simulink model "ThdRwLtStFwdBkwdCtrl"  (R2024b)
settings: Solver=FixedStepDiscrete  StartTime=0.0  StopTime=10.0  FixedStep=0.01  RelTol=1e-3
undefined symbols (not defined in the file or in its folder): KeSMSuMdMotFinshdTm_Val, KeSMSuMdRetryTm1_Val, KeSMSuModeReqDurgTm_Val, KeSMSwThdRwLtStFwdBkwdEnTrigBitMask6s_Val, KeSMSwThdRwLtStFwdBkwdEnTrigBitMask_Val
libraries: StCtrlLibBkRecln x1
settings Model: ModifiedHistory=24.6.21 V2.4.0 557模式流程V1.6  Creator=sn2xws  LastModifiedBy=sn55gm
settings SolverCC: AlgebraicLoopSolver=TrustRegion
settings DataIOCC: SaveFormat=StructureWithTime  ReturnWorkspaceOutputs=off
settings OptimizationCC: DefaultParameterBehavior=Inlined  EnhancedBackFolding=on  PassReuseOutputArgsAs=Individual arguments  ZeroExternalMemoryAtStartup=off  ZeroInternalMemoryAtStartup=off  OptimizeBlockOrder=speed  DifferentSizesBufferReuse=on  OptimizationCustomize=off  EfficientTunableParamExpr=on
settings DebuggingCC: ParameterTunabilityLossMsg=error  UnconnectedInputMsg=warning  UnconnectedOutputMsg=warning  UnconnectedLineMsg=warning  ArithmeticOperatorsInVariantConditions=warning
settings ModelReferenceCC: EnableRefExpFcnMdlSchedulingChecks=on  ModelReferenceNumInstancesAllowed=Single
settings SFSimCC: MATLABDynamicMemAlloc=off  CustomCodeUndefinedFunction=UseInterfaceOnly
settings RTWCC: Description=AUTOSAR  SystemTargetFile=autosar.tlc  GenCodeOnly=on  TemplateMakefile=ert_default_tmf  GenerateReport=on  IncludeHyperlinkInReport=on  LaunchReport=on  DataTypeReplacement=CDataTypesFixedWidth  GenerateTraceInfo=on  GenerateTraceReport=on  GenerateTraceReportSl=on  GenerateTraceReportSf=on  GenerateTraceReportEml=on  GPUComputeCapability=3.5
settings CodeAppCC: ForceParamTrailComments=on  IgnoreCustomStorageClasses=off  OperatorAnnotations=on  SimulinkDataObjDesc=on  SFDataObjDesc=on  InsertBlockDesc=on
settings STFCustomTargetCC: TargetLangStandard=C99 (ISO)  MultiwordLength=256  ParMdlRefBuildCompliant=on  CompOptLevelCompliant=on  IncludeMdlTerminateFcn=off  CombineOutputUpdateFcns=on  SuppressErrorStatus=on  ERTCustomFileBanners=on  SupportNonFinite=off  SupportComplex=off  SupportContinuousTime=off  SupportNonInlinedSFcns=off  RemoveResetFunc=on  MATLABClassNameForMDSCustomization=Simulink.SoftwareTarget.ERTCustomization  AutosarCompliant=on  UseToolchainInfoCompliant=on  LookupTableObjectStructAxisOrder=2,1,3,4,...  LUTObjectStructOrderEvenSpacing=Size,Table,Breakpoints  SystemTargetFile=autosar.tlc
settings ERTTargetCC: TargetLangStandard=C99 (ISO)  ConcurrentExecutionCompliant=off  IncludeMdlTerminateFcn=off  SuppressErrorStatus=on  SupportNonFinite=off  SupportComplex=off  ModelStepFunctionPrototypeControlCompliant=off  CPPClassGenCompliant=off  AutosarCompliant=on  LookupTableObjectStructAxisOrder=2,1,3,4,...  LUTObjectStructOrderEvenSpacing=Size,Table,Breakpoints  ERTCustomFileTemplate=example_file_process.tlc  ERTFilePackagingFormat=Compact  BooleanTrueId=TRUE  BooleanFalseId=FALSE  DynamicArrayContainerType=coder::array

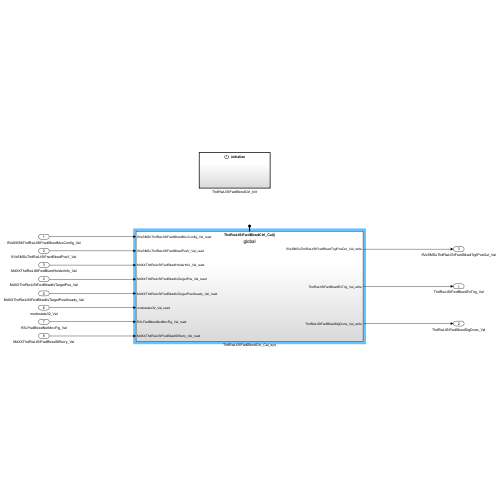
[thumbnail: Simulink's stored preview of the top-level diagram]
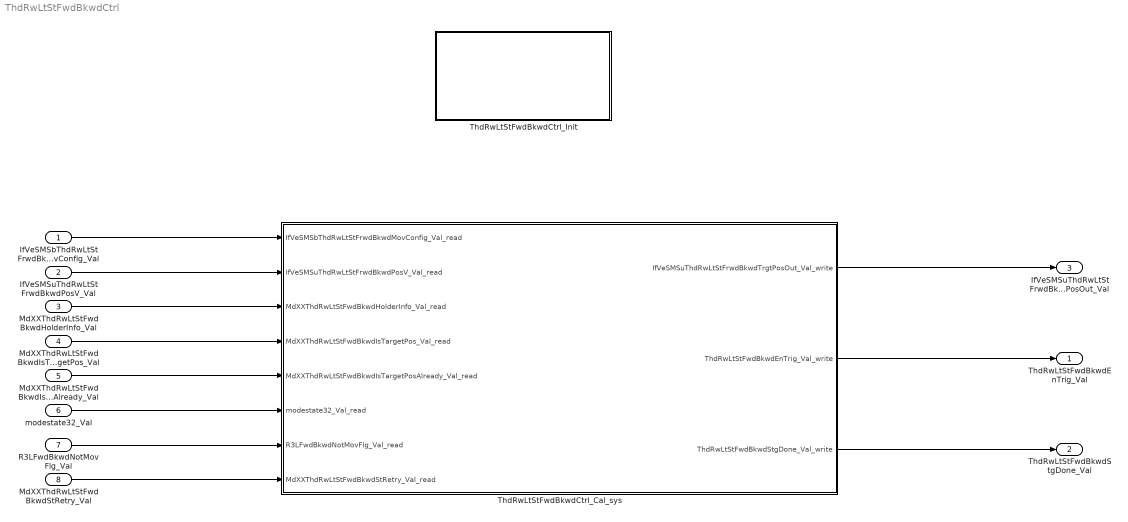
== system ThdRwLtStFwdBkwdCtrl ==
  IfVeSMSbThdRwLtStFrwdBkwdMovConfig_Val : Inport  OutDataTypeStr=boolean  PortDimensions=1
  IfVeSMSuThdRwLtStFrwdBkwdPosV_Val : Inport  Port=2  OutDataTypeStr=boolean  PortDimensions=1
  MdXXThdRwLtStFwdBkwdHolderInfo_Val : Inport  Port=3  OutDataTypeStr=uint32  PortDimensions=1
  MdXXThdRwLtStFwdBkwdIsTargetPos_Val : Inport  Port=4  OutDataTypeStr=uint32  PortDimensions=1
  MdXXThdRwLtStFwdBkwdIsTargetPosAlready_Val : Inport  Port=5  OutDataTypeStr=uint32  PortDimensions=1
  modestate32_Val : Inport  Port=6  OutDataTypeStr=uint32  PortDimensions=1
  R3LFwdBkwdNotMovFlg_Val : Inport  Port=7  OutDataTypeStr=boolean  PortDimensions=1
  MdXXThdRwLtStFwdBkwdStRetry_Val : Inport  Port=8  OutDataTypeStr=uint32  PortDimensions=1
  ThdRwLtStFwdBkwdCtrl_Cal_sys : Subsystem
  ThdRwLtStFwdBkwdCtrl_Init : Subsystem
  ThdRwLtStFwdBkwdEnTrig_Val : Outport  OutDataTypeStr=boolean  PortDimensions=1  VectorParamsAs1DForOutWhenUnconnected=off
  ThdRwLtStFwdBkwdStgDone_Val : Outport  Port=2  OutDataTypeStr=boolean  PortDimensions=1  VectorParamsAs1DForOutWhenUnconnected=off
  IfVeSMSuThdRwLtStFrwdBkwdTrgtPosOut_Val : Outport  Port=3  OutDataTypeStr=boolean  PortDimensions=1  VectorParamsAs1DForOutWhenUnconnected=off
  wires:
  IfVeSMSbThdRwLtStFrwdBkwdMovConfig_Val/1 -> ThdRwLtStFwdBkwdCtrl_Cal_sys/1(IfVeSMSbThdRwLtStFrwdBkwdMovConfig_Val_read)
  IfVeSMSuThdRwLtStFrwdBkwdPosV_Val/1 -> ThdRwLtStFwdBkwdCtrl_Cal_sys/2(IfVeSMSuThdRwLtStFrwdBkwdPosV_Val_read)
  MdXXThdRwLtStFwdBkwdHolderInfo_Val/1 -> ThdRwLtStFwdBkwdCtrl_Cal_sys/3(MdXXThdRwLtStFwdBkwdHolderInfo_Val_read)
  MdXXThdRwLtStFwdBkwdIsTargetPos_Val/1 -> ThdRwLtStFwdBkwdCtrl_Cal_sys/4(MdXXThdRwLtStFwdBkwdIsTargetPos_Val_read)
  MdXXThdRwLtStFwdBkwdIsTargetPosAlready_Val/1 -> ThdRwLtStFwdBkwdCtrl_Cal_sys/5(MdXXThdRwLtStFwdBkwdIsTargetPosAlready_Val_read)
  modestate32_Val/1 -> ThdRwLtStFwdBkwdCtrl_Cal_sys/6(modestate32_Val_read)
  R3LFwdBkwdNotMovFlg_Val/1 -> ThdRwLtStFwdBkwdCtrl_Cal_sys/7(R3LFwdBkwdNotMovFlg_Val_read)
  ThdRwLtStFwdBkwdCtrl_Cal_sys/1(IfVeSMSuThdRwLtStFrwdBkwdTrgtPosOut_Val_write) -> IfVeSMSuThdRwLtStFrwdBkwdTrgtPosOut_Val/1
  ThdRwLtStFwdBkwdCtrl_Cal_sys/2(ThdRwLtStFwdBkwdEnTrig_Val_write) -> ThdRwLtStFwdBkwdEnTrig_Val/1
  ThdRwLtStFwdBkwdCtrl_Cal_sys/3(ThdRwLtStFwdBkwdStgDone_Val_write) -> ThdRwLtStFwdBkwdStgDone_Val/1
  MdXXThdRwLtStFwdBkwdStRetry_Val/1 -> ThdRwLtStFwdBkwdCtrl_Cal_sys/8(MdXXThdRwLtStFwdBkwdStRetry_Val_read)

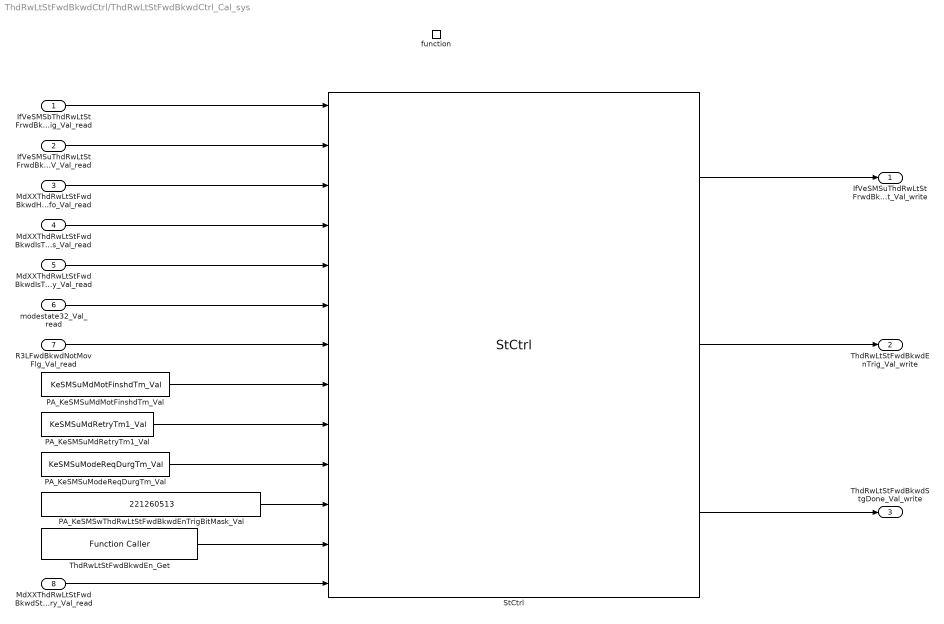
== system ThdRwLtStFwdBkwdCtrl/ThdRwLtStFwdBkwdCtrl_Cal_sys ==
  IfVeSMSbThdRwLtStFrwdBkwdMovConfig_Val_read : Inport
  IfVeSMSuThdRwLtStFrwdBkwdPosV_Val_read : Inport  Port=2
  MdXXThdRwLtStFwdBkwdHolderInfo_Val_read : Inport  Port=3
  MdXXThdRwLtStFwdBkwdIsTargetPos_Val_read : Inport  Port=4
  MdXXThdRwLtStFwdBkwdIsTargetPosAlready_Val_read : Inport  Port=5
  modestate32_Val_read : Inport  Port=6
  R3LFwdBkwdNotMovFlg_Val_read : Inport  Port=7
  MdXXThdRwLtStFwdBkwdStRetry_Val_read : Inport  Port=8
  function : TriggerPort  TriggerType=function-call  IsSimulinkFunction=on  FunctionName=ThdRwLtStFwdBkwdCtrl_Cal  VariantControl=(inherit)
  PA_KeSMSuMdMotFinshdTm_Val : Constant  Value=KeSMSuMdMotFinshdTm_Val
  PA_KeSMSuMdRetryTm1_Val : Constant  Value=KeSMSuMdRetryTm1_Val
  PA_KeSMSuModeReqDurgTm_Val : Constant  Value=KeSMSuModeReqDurgTm_Val
  PA_KeSMSwThdRwLtStFwdBkwdEnTrigBitMask_Val : Constant  Value=221260513  OutDataTypeStr=uint32
  StCtrl : StCtrlLibBkRecln/StCtrl  SystemSampleTime=-1  VariantActivationTime=update diagram  AllowFlexibleInterface=on  Latency=0  AutoFrameSizeCalculation=off
  ThdRwLtStFwdBkwdEn_Get : FunctionCaller  FunctionPrototype=data = ThdRwLtStFwdBkwdEn_Get()  InputArgumentSpecifications=<Enter example>  OutputArgumentSpecifications=uint32(1)
  IfVeSMSuThdRwLtStFrwdBkwdTrgtPosOut_Val_write : Outport  VectorParamsAs1DForOutWhenUnconnected=off
      settings: EnsureOutportIsVirtual=on
  ThdRwLtStFwdBkwdEnTrig_Val_write : Outport  Port=2  VectorParamsAs1DForOutWhenUnconnected=off
      settings: EnsureOutportIsVirtual=on
  ThdRwLtStFwdBkwdStgDone_Val_write : Outport  Port=3  VectorParamsAs1DForOutWhenUnconnected=off
      settings: EnsureOutportIsVirtual=on
  wires:
  StCtrl/1 -> IfVeSMSuThdRwLtStFrwdBkwdTrgtPosOut_Val_write/1
  StCtrl/2 -> ThdRwLtStFwdBkwdEnTrig_Val_write/1
  StCtrl/3 -> ThdRwLtStFwdBkwdStgDone_Val_write/1
  PA_KeSMSuMdMotFinshdTm_Val/1 -> StCtrl/8
  ThdRwLtStFwdBkwdEn_Get/1 -> StCtrl/12
  PA_KeSMSuModeReqDurgTm_Val/1 -> StCtrl/10
  PA_KeSMSuMdRetryTm1_Val/1 -> StCtrl/9
  IfVeSMSbThdRwLtStFrwdBkwdMovConfig_Val_read/1 -> StCtrl/1
  IfVeSMSuThdRwLtStFrwdBkwdPosV_Val_read/1 -> StCtrl/2
  MdXXThdRwLtStFwdBkwdHolderInfo_Val_read/1 -> StCtrl/3
  MdXXThdRwLtStFwdBkwdIsTargetPos_Val_read/1 -> StCtrl/4
  MdXXThdRwLtStFwdBkwdIsTargetPosAlready_Val_read/1 -> StCtrl/5
  modestate32_Val_read/1 -> StCtrl/6
  R3LFwdBkwdNotMovFlg_Val_read/1 -> StCtrl/7
  MdXXThdRwLtStFwdBkwdStRetry_Val_read/1 -> StCtrl/13
  PA_KeSMSwThdRwLtStFwdBkwdEnTrigBitMask_Val/1 -> StCtrl/11

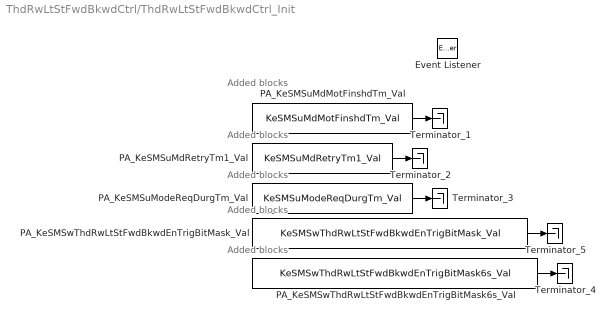
== system ThdRwLtStFwdBkwdCtrl/ThdRwLtStFwdBkwdCtrl_Init ==
  note: Added blocks
  note: Added blocks
  note: Added blocks
  note: Added blocks
  note: Added blocks
  Event Listener : EventListener  EventName=reset
  PA_KeSMSuMdMotFinshdTm_Val : Constant  Value=KeSMSuMdMotFinshdTm_Val
  PA_KeSMSuMdRetryTm1_Val : Constant  Value=KeSMSuMdRetryTm1_Val
  PA_KeSMSuModeReqDurgTm_Val : Constant  Value=KeSMSuModeReqDurgTm_Val
  PA_KeSMSwThdRwLtStFwdBkwdEnTrigBitMask6s_Val : Constant  Value=KeSMSwThdRwLtStFwdBkwdEnTrigBitMask6s_Val
  PA_KeSMSwThdRwLtStFwdBkwdEnTrigBitMask_Val : Constant  Value=KeSMSwThdRwLtStFwdBkwdEnTrigBitMask_Val
  Terminator_{1..5} (5 alike) : Terminator
  wires:
  PA_KeSMSuMdMotFinshdTm_Val/1 -> Terminator_1/1
  PA_KeSMSuMdRetryTm1_Val/1 -> Terminator_2/1
  PA_KeSMSuModeReqDurgTm_Val/1 -> Terminator_3/1
  PA_KeSMSwThdRwLtStFwdBkwdEnTrigBitMask6s_Val/1 -> Terminator_4/1
  PA_KeSMSwThdRwLtStFwdBkwdEnTrigBitMask_Val/1 -> Terminator_5/1
